simulink subsystem "posture_subsys"  (R2022b)
settings: Solver=VariableStepAuto  StartTime=0.0  StopTime=10.0  RelTol=1e-3
model mask{InitialCondition=initial_conditions_trans}
  mask prompts: InitialCondition "Simulink:blkprm_prompts:IntegratorInitCond"
settings Model: Creator=Edp  LastModifiedBy=Edp

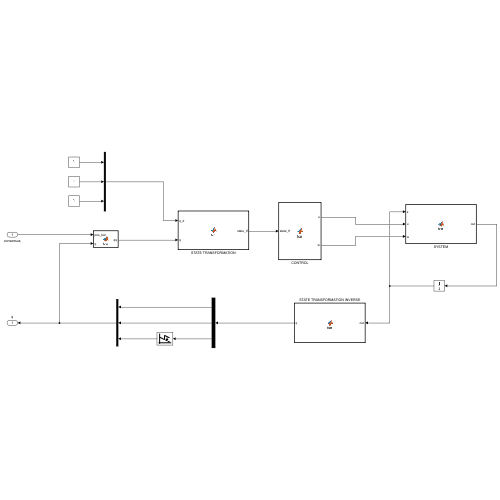
[thumbnail: Simulink's stored preview of the top-level diagram]
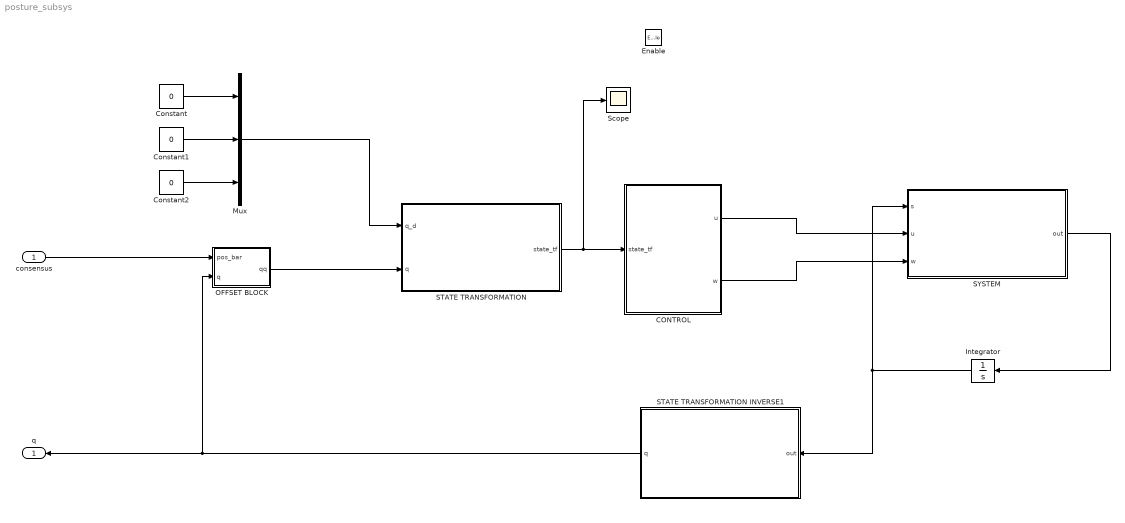
== system posture_subsys ==
  consensus : Inport
  Enable : EnablePort
  CONTROL : MATLAB Function  TreatAsAtomicUnit=on
  Constant : Constant  Value=0
  Constant1 : Constant  Value=0
  Constant2 : Constant  Value=0
  Integrator : Integrator  InitialCondition=InitialCondition
  Mux : Mux  Inputs=3
  OFFSET BLOCK : MATLAB Function  TreatAsAtomicUnit=on
  STATE TRANSFORMATION : MATLAB Function  TreatAsAtomicUnit=on
  STATE TRANSFORMATION INVERSE1 : MATLAB Function  TreatAsAtomicUnit=on
  SYSTEM : MATLAB Function  TreatAsAtomicUnit=on
  Scope : Scope
  q : Outport
  wires:
  Mux/1 -> STATE TRANSFORMATION/1(q_d)
  STATE TRANSFORMATION/1(state_tf) -> CONTROL/1(state_tf), Scope/1
  CONTROL/1(u) -> SYSTEM/2(u)
  Constant1/1 -> Mux/2
  Constant2/1 -> Mux/3
  SYSTEM/1(out) -> Integrator/1
  Integrator/1 -> SYSTEM/1(s), STATE TRANSFORMATION INVERSE1/1(out)
  CONTROL/2(w) -> SYSTEM/3(w)
  Constant/1 -> Mux/1
  consensus/1 -> OFFSET BLOCK/1(pos_bar)
  STATE TRANSFORMATION INVERSE1/1(q) -> q/1, OFFSET BLOCK/2(q)
  OFFSET BLOCK/1(qq) -> STATE TRANSFORMATION/2(q)

== matlab function posture_subsys/CONTROL ==
  data: state_tf input; u output; w output
function [u, w]= fcn(state_tf)
k1 = 1;
k2 = 20;
k3 = 2*k1;

rho = state_tf(1);
gamma = state_tf(2);
delta = state_tf(3);

u = k1 * rho * cos(gamma);
w = k2 * gamma + k1*sin(gamma)*cos(gamma)/gamma*(gamma + k3*delta);

== matlab function posture_subsys/OFFSET BLOCK ==
  data: pos_bar input; qq output; q input
function qq = fcn(pos_bar, q)
qq = [0, 0, 0];
qq(1) = q(1) - pos_bar(1);
qq(2) = q(2) - pos_bar(2);
qq(3) = q(3);

== matlab function posture_subsys/STATE TRANSFORMATION ==
  data: q_d input; state_tf output; q input
function state_tf = fcn(q_d, q)

x = q(1);
y = q(2);
theta = q(3);

rho = sqrt(x^2 + y^2);
gamma = mod(atan2(y,x),2*pi) + pi - theta;
delta = gamma + theta;

state_tf = [rho, gamma, delta];

== matlab function posture_subsys/STATE TRANSFORMATION INVERSE1 ==
  data: out input; q output
function q = fcn(out)

rho = out(1);
gamma = out(2);
delta = out(3);

q = [0, 0, 0];
q(1) = -rho*cos(delta);
q(2) = -rho*sin(delta);
q(3) = delta - gamma;

== matlab function posture_subsys/SYSTEM ==
  data: s input; out output; u input; w input
function out = fcn(s, u, w)

rd = -s(1)*u*cos(s(2));
gd = u*sin(s(2)) - w;
dd = u*sin(s(2));

out = [rd, gd, dd];
